simulink model "TwoTanks"  (R2018b)
settings: Solver=VariableStepAuto  StartTime=0.0  StopTime=10.0  RelTol=1e-3
settings Model: Creator=root  LastModifiedBy=root

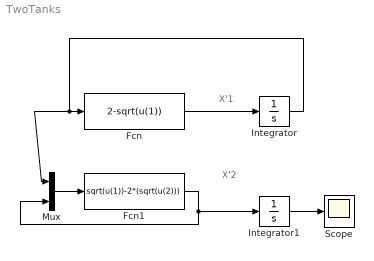
== system TwoTanks ==
  note: X'2
  note: X'1
  Fcn : Fcn  Expr=2-sqrt(u(1))
  Fcn1 : Fcn  Expr=sqrt(u(1))-2*(sqrt(u(2)))
  Integrator : Integrator  InitialCondition=0.1
  Integrator1 : Integrator  InitialCondition=0.1
  Mux : Mux  Inputs=2
  Scope : Scope
  wires:
  Fcn/1 -> Integrator/1
  Fcn1/1 -> Integrator1/1, Mux/2
  Integrator/1 -> Mux/1, Fcn/1
  Mux/1 -> Fcn1/1
  Integrator1/1 -> Scope/1
